simulink model "lab6"  (R2017b)
settings: Solver=ode4  StartTime=0.0  StopTime=100  FixedStep=0.0001  RelTol=1e-3
undefined symbols (not defined in the file or in its folder): b, k, m1, m2
settings Model: Creator=ayushi  LastModifiedBy=ayushi

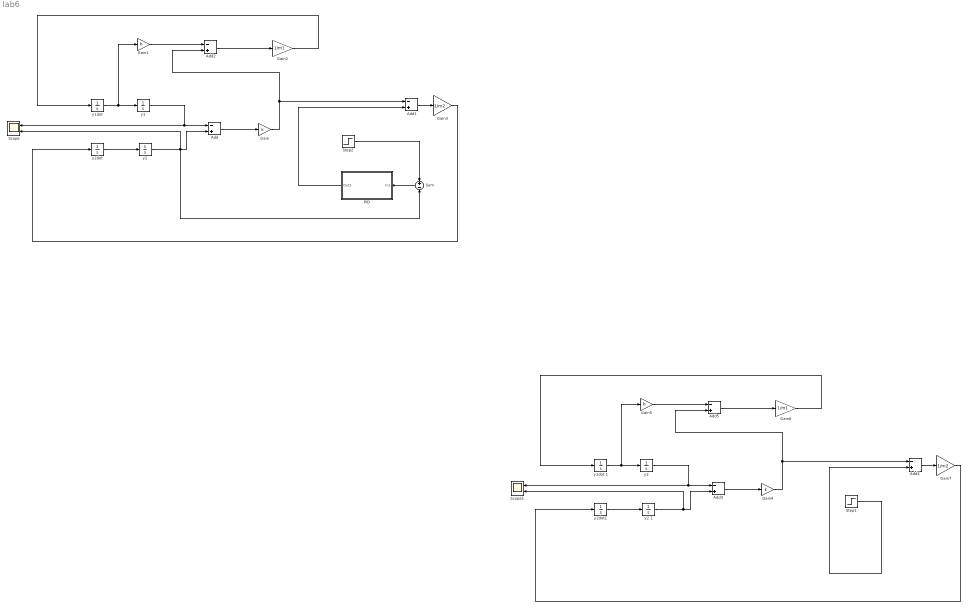
== system lab6 ==
  Add{,1..5} (6 alike) : Sum  Inputs=-+
  Gain : Gain  Gain=k
  Gain1 : Gain  Gain=b
  Gain2 : Gain  Gain=1/m1
  Gain3 : Gain  Gain=1/m2
  Gain4 : Gain  Gain=k
  Gain5 : Gain  Gain=b
  Gain6 : Gain  Gain=1/m1
  Gain7 : Gain  Gain=1/m2
  "PID " : Subsystem
  Scope : Scope  NumInputPorts=2
  Scope1 : Scope  NumInputPorts=2
  Step1 : Step  SampleTime=0
  Step2 : Step  SampleTime=0
  Sum : Sum  Inputs=+-
  y1 : Integrator
  "y1dot " : Integrator
  y1dot 1 : Integrator
  y2 : Integrator
  "y2 " : Integrator
  y2 1 : Integrator
  y2dot : Integrator
  y2dot1 : Integrator
  wires:
  Add1/1 -> Gain3/1
  y2dot/1 -> "y2 "/1
  "y1dot "/1 -> Gain1/1, y1/1
  y1/1 -> Add/1, Scope/1
  "y2 "/1 -> Add/2, Scope/2, Sum/2
  Gain/1 -> Add1/1, Add2/2
  Gain1/1 -> Add2/1
  Add/1 -> Gain/1
  Add2/1 -> Gain2/1
  Gain2/1 -> "y1dot "/1
  Gain3/1 -> y2dot/1
  Step2/1 -> Sum/1
  Sum/1 -> "PID "/1(In1)
  "PID "/1(Out1) -> Add1/2
  Add3/1 -> Gain4/1
  y2/1 -> Add3/1, Scope1/1
  y2 1/1 -> Add3/2, Scope1/2
  Gain6/1 -> y1dot 1/1
  Gain5/1 -> Add5/1
  Add5/1 -> Gain6/1
  Gain4/1 -> Add4/1, Add5/2
  y2dot1/1 -> y2 1/1
  Add4/1 -> Gain7/1
  Gain7/1 -> y2dot1/1
  y1dot 1/1 -> Gain5/1, y2/1
  Step1/1 -> Add4/2

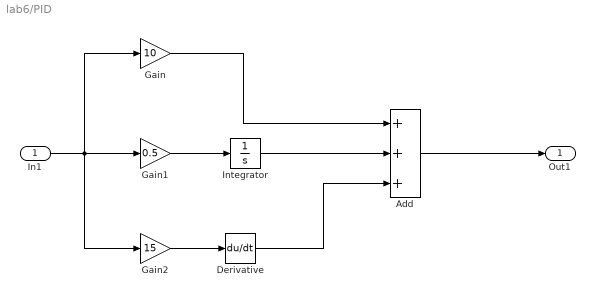
== system lab6/PID  ==
  In1 : Inport
  Add : Sum  Inputs=+++
  Derivative : Derivative
  Gain : Gain  Gain=10
  Gain1 : Gain  Gain=0.5
  Gain2 : Gain  Gain=15
  Integrator : Integrator
  Out1 : Outport
  wires:
  Gain/1 -> Add/1
  Gain2/1 -> Derivative/1
  Derivative/1 -> Add/3
  Integrator/1 -> Add/2
  Add/1 -> Out1/1
  In1/1 -> Gain2/1, Gain/1, Gain1/1
  Gain1/1 -> Integrator/1
